simulink model "semplificato"  (R2023b)
settings: Solver=VariableStepAuto  StartTime=0.0  StopTime=10.0  RelTol=1e-3
values from neighbouring files (symbols this model uses):
  m = 1    [main_feedback_lin.m]
undefined symbols (not defined in the file or in its folder): k_aero, k_mag_mod, Lc_mod, Rtot_mod, theta, y0
settings Model: Creator=lollo  LastModifiedBy=lollo

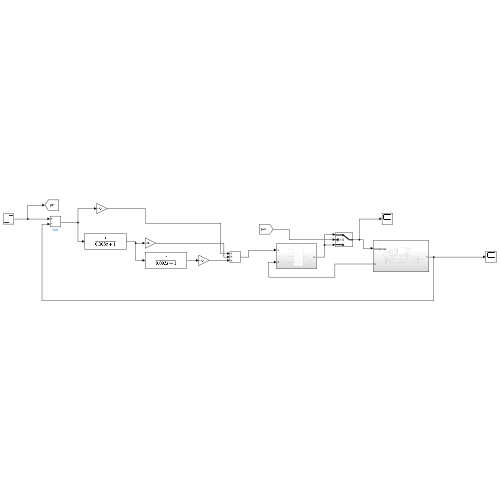
[thumbnail: Simulink's stored preview of the top-level diagram]
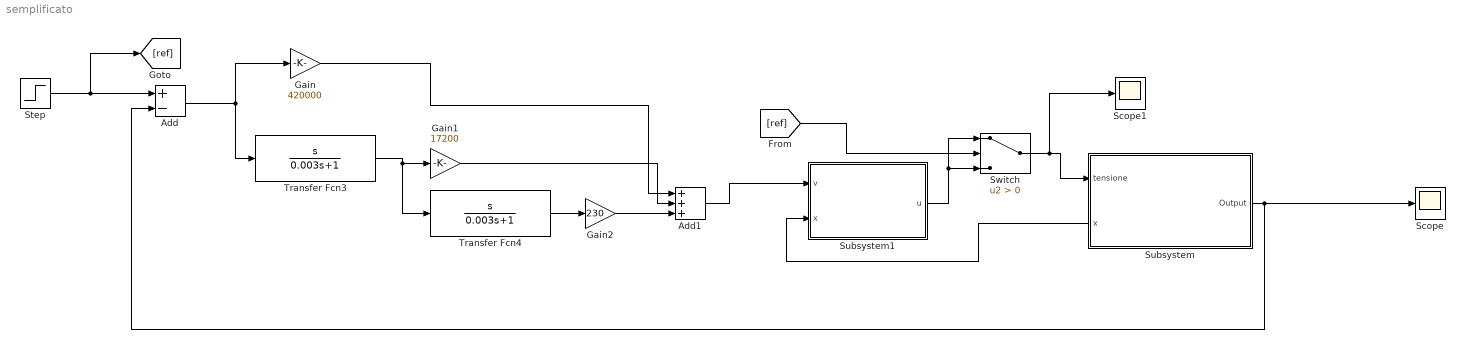
== system semplificato ==
  Add : Sum  Inputs=+-
  Add1 : Sum  Inputs=+++
  Gain : Gain  Gain=420000
  Gain1 : Gain  Gain=17200
  Gain2 : Gain  Gain=230
  Scope : Scope
  Scope1 : Scope
  Step : Step  After=0.004  SampleTime=0
  Subsystem : Subsystem
      settings: PortSchema="{\"entries\":[{\"content\":{\"sides\":[{\"content\":{\"connectorIds\":[\"In1\",\"Out2\"]},\"type\":\"ConnectorPlacement.EquallySpacedRectSide\",\"uuid\":\"aaa18915-a376-47c2-b377-85246a10492a\"},{\"content\":{\"connectorIds\":[\"Out1\"],\"side\":\"RIGHT\"},\"type\":\"ConnectorPlacement.EquallySpacedRectSide\",\"uuid\":\"11739fae-64b3-4756-9522-de4aa171849c\"},{\"content\":{\"side\":\"TOP\"},\"type\":\"ConnectorPlacement.EquallySpacedRectSide\",\"uuid\":\"71f42e56-43d1-4921-85cf-46a38dfcc470\"}]},\"type\":\"ConnectorPlacement.EquallySpacedConnector\",\"uuid\":\"c3819c32-ee1c-47d4-b1ba-004038871bfd\"}],\"packageUris\":[\"http://schema.mathworks.com/mf0/Connector/R2020b\"],\"version\":\"1.0\"}"
  Subsystem1 : Subsystem
  Switch : Switch  Criteria=u2 > Threshold  SaturateOnIntegerOverflow=off  InputSameDT=off
  Transfer Fcn3 : TransferFcn  Numerator=[1 0]  Denominator=[0.003 1]
  Transfer Fcn4 : TransferFcn  Numerator=[1 0]  Denominator=[0.003 1]
  wires:
  Step/1 -> [ref], Add/1
  Gain/1 -> Add1/1
  Add/1 -> Transfer Fcn3/1, Gain/1
  Gain1/1 -> Add1/2
  Transfer Fcn3/1 -> Gain1/1, Transfer Fcn4/1
  Transfer Fcn4/1 -> Gain2/1
  Gain2/1 -> Add1/3
  Add1/1 -> Subsystem1/1(v)
  Subsystem/1(Output) -> Add/2, Scope/1
  Subsystem1/1(u) -> Switch/1, Switch/3
  Subsystem/2(x) -> Subsystem1/2(x)
  [ref] -> Switch/2
  Switch/1 -> Scope1/1, Subsystem/1(tensione)

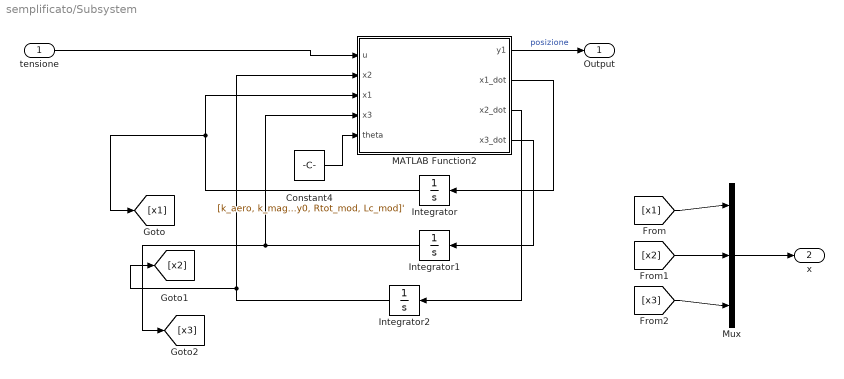
== system semplificato/Subsystem ==
  tensione : Inport
  Constant4 : Constant  Value=[k_aero, k_mag_mod, m, y0, Rtot_mod, Lc_mod]'
  Integrator : Integrator
  Integrator1 : Integrator
  Integrator2 : Integrator
  MATLAB Function2 : MATLAB Function  TreatAsAtomicUnit=on
  Mux : Mux  Inputs=3
  Output : Outport
  x : Outport  Port=2
  wires:
  Constant4/1 -> MATLAB Function2/5(theta)
  Integrator1/1 -> [x3], MATLAB Function2/4(x3)
  MATLAB Function2/3(x2_dot) -> Integrator2/1
  tensione/1 -> MATLAB Function2/1(u)
  Integrator/1 -> [x1], MATLAB Function2/3(x1)
  MATLAB Function2/1(y1) -> Output/1  "posizione"
  MATLAB Function2/2(x1_dot) -> Integrator/1
  MATLAB Function2/4(x3_dot) -> Integrator1/1
  Integrator2/1 -> [x2], MATLAB Function2/2(x2)
  Mux/1 -> x/1
  [x1] -> Mux/1
  [x2] -> Mux/2
  [x3] -> Mux/3

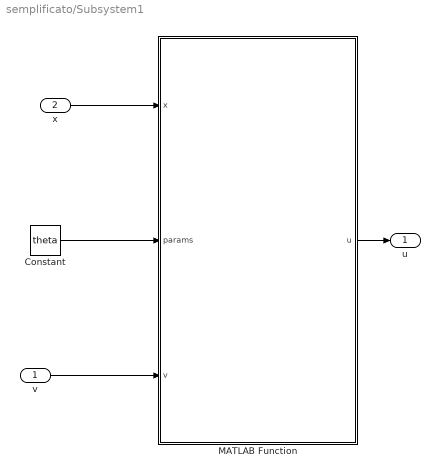
== system semplificato/Subsystem1 ==
  v : Inport
  x : Inport  Port=2
  Constant : Constant  Value=theta
  MATLAB Function : MATLAB Function  TreatAsAtomicUnit=on
  u : Outport
  wires:
  v/1 -> MATLAB Function/3(v)
  MATLAB Function/1(u) -> u/1
  Constant/1 -> MATLAB Function/2(params)
  x/1 -> MATLAB Function/1(x)

== matlab function semplificato/Subsystem1/MATLAB Function ==
  data: x input; u output; params input; v input
function u  = feedback_linearization_control(x, params, v)
    % Estrai parametri
    k_aero = params(1);
    k_mag  = params(2);
    m      = params(3);
    y0     = params(4);
    Rtot   = params(5);
    Lc     = params(6);
    g      = 9.81;

    % Stati
    x1 = x(1); % posizione
    x2 = x(2); % corrente
    x3 = x(3); % velocità

    % Derivate
    denom = (y0 - x1);
    if denom <= 0
        warning('Denominatore nullo o negativo: instabilità elettromagnetica');
    end

    % Accelerazione reale
    xdot3 = (k_aero/m)*x3 + (k_mag/m)*(x2 / denom)^2 - g;

    % Derivate parziali
    dBdx1 = (2 * k_mag * x2^2) / (m * denom^3);
    dBdx2 = (2 * k_mag * x2)   / (m * denom^2);
    dBdx3 = (k_aero/m);

    % Corrente senza ingresso (per calcolo alpha)
    dx2_nou = -(Rtot/Lc)*x2;

    % Parte non lineare (α) e lineare (β)
    alpha = dBdx1 * x3 + dBdx2 * dx2_nou + dBdx3 * xdot3;
    beta  = dBdx2 * (1/Lc);

    if abs(beta) < 1e-6
        warning('Beta troppo piccolo: possibile instabilità numerica');
        u = 5;
        return;
    end


    % Controllo reale
    u = (v - alpha) / beta;
end

== matlab function semplificato/Subsystem/MATLAB Function2 ==
  data: u input; y1 output; x2 input; x1_dot output; x2_dot output; x1 input; x3 input; x3_dot output; theta input
function [y1,x1_dot, x2_dot, x3_dot] = fcn(u, x2, x1, x3, theta)
    k_aero = theta(1, 1);
    k_mag = theta(2, 1);
    m = theta(3, 1);
    y0 = theta(4, 1);
    Rtot = theta(5, 1);
    Lc = theta(6, 1);
    g = 9.81;
    
    x2_dot = 1/Lc*(-Rtot*x2 + u);

    x1_dot = x3;
    x3_dot = (k_mag/m)*(x2/(y0-x1))^2 - g;
    % if x1 < y0
    %     x3_dot = (k_mag/m)*(x2/(y0-x1))^2 - g;
    % else
    %     x1 = 0.012;
    %     x3_dot = 0;
    %     x3 = 0;
    % end
    % 
    % 
    % % condizioni
    % if x1 <=0 && x3_dot < 0
    %     x1 = 0;
    %     x3 = 0;
    %     x3_dot = 0;
    % end
y1 = x1;
